simulink model "sideslip_hold"  (Simulink 7.7)
settings: Solver=ode45  StartTime=0.0  StopTime=10.0  RelTol=1e-3
undefined symbols (not defined in the file): a_beta_1, a_beta_2, k_i_beta, k_p_beta
settings Model: Creator=prattmic  LastModifiedBy=prattmic

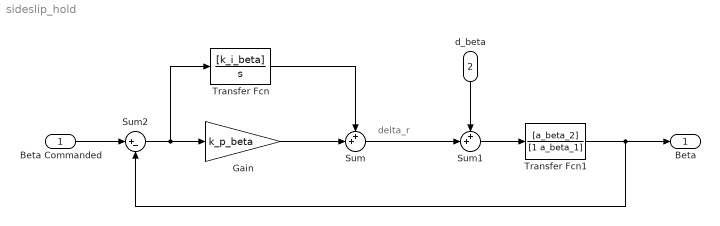
== system sideslip_hold ==
  note: delta_r
  Beta Commanded : Inport
  d_beta : Inport  Port=2
  Gain : Gain  Gain=k_p_beta
  Sum : Sum  Inputs=++|
  Sum1 : Sum  Inputs=++|
  Sum2 : Sum  Inputs=|+-
  Transfer Fcn : TransferFcn  Numerator=[k_i_beta]  Denominator=[1 0]
  Transfer Fcn1 : TransferFcn  Numerator=[a_beta_2]  Denominator=[1 a_beta_1]
  Beta : Outport
  wires:
  d_beta/1 -> Sum1/1
  Transfer Fcn/1 -> Sum/1
  Gain/1 -> Sum/2
  Sum/1 -> Sum1/2
  Sum1/1 -> Transfer Fcn1/1
  Transfer Fcn1/1 -> Beta/1, Sum2/2
  Sum2/1 -> Gain/1, Transfer Fcn/1
  Beta Commanded/1 -> Sum2/1
